simulink model "model_graphicSim_OnlyDist"  (R2022a)
settings: Solver=FixedStepAuto  StartTime=0.0  StopTime=inf  RelTol=1e-3
values from neighbouring files (symbols this model uses):
  A = 3*3    (= 9)    [Configuration.m]    (also in test_sim.mat; test_sim_10000Ep_v10.mat; test_sim_10000Ep_v12_G_oldScen.mat; test_sim_10000Ep_v1_dist.mat)
  d = A*N*nCells    (= 699840)    [Configuration.m]    (also in get_features.m = A*N*nCells; test_sim.mat = 18432; test_sim_10000Ep_v10.mat; test_sim_10000Ep_v12_G_oldScen.mat)
  egoID = 1    [Configuration.m]    (also in test_sim.mat; test_sim_10000Ep_v10.mat; test_sim_10000Ep_v12_G_oldScen.mat; test_sim_10000Ep_v1_dist.mat)
  frontDistCG = 3.7    [Configuration.m]    (also in test_sim_10000Ep_v10.mat; test_sim_10000Ep_v12_G_oldScen.mat; test_sim_10000Ep_v1_dist.mat; test_sim_1000Ep.mat)
  gridvx = zeros(N, length(TVX))    [construct_tiles.m]    (also in test_sim.mat = [-3.33333333333 -3.21428571429 -3.09523809524 -2.97619047619; test_sim_10000Ep_v10.mat = [-2.8 -2.75555555556 -2.71111111111 -2.66666666667 -2.622222; test_sim_10000Ep_v12_G_oldScen.mat = [-2.8 -2.75555555556 -2.71111111111 -2.66666666667 -2.622222; test_sim_10000Ep_v1_dist.mat = [-2.8 -2.75555555556 -2.71111111111 -2.66666666667 -2.622222)
  gridvy = zeros(N, length(TVY))    [construct_tiles.m]    (also in test_sim.mat = [-3.33333333333 -3.16666666667 -3 -2.83333333333 -2.66666666; test_sim_10000Ep_v10.mat = [-28 -27.3777777778 -26.7555555556 -26.1333333333 -25.511111; test_sim_10000Ep_v12_G_oldScen.mat = [-28 -27.3777777778 -26.7555555556 -26.1333333333 -25.511111; test_sim_10000Ep_v1_dist.mat = [-28 -27.3777777778 -26.7555555556 -26.1333333333 -25.511111)
  gridx = zeros(N, length(TX))    [construct_tiles.m]    (also in test_sim.mat = [-8.33333333333 -8.18452380952 -8.03571428571 -7.8869047619 ; test_sim_10000Ep_v10.mat = [-5 -4.94444444444 -4.88888888889 -4.83333333333 -4.77777777; test_sim_10000Ep_v12_G_oldScen.mat = [-5 -4.94444444444 -4.88888888889 -4.83333333333 -4.77777777; test_sim_10000Ep_v1_dist.mat = [-5 -4.94444444444 -4.88888888889 -4.83333333333 -4.77777777)
  gridy = zeros(N, length(TY))    [construct_tiles.m]    (also in test_sim.mat = [-16.6666666667 -16.3095238095 -15.9523809524 -15.5952380952; test_sim_10000Ep_v10.mat = [-2 -1.93333333333 -1.86666666667 -1.8 -1.73333333333 -1.666; test_sim_10000Ep_v12_G_oldScen.mat = [-2 -1.93333333333 -1.86666666667 -1.8 -1.73333333333 -1.666; test_sim_10000Ep_v1_dist.mat = [0.4 0.453333333333 0.506666666667 0.56 0.613333333333 0.666)
  gridyaw = [-504 -489.6 -475.2 -460.8 -446.4 -432 -417.6 -403.2 -388.8 -374.4 -360 -345.6 ... (70 elements, 10x7)]    [test_sim_10000Ep_v10.mat]    (also in test_sim_10000Ep_v12_G_oldScen.mat; test_sim_10000Ep_v1_dist.mat = [-126 -122.4 -118.8 -115.2 -111.6 -108 -104.4 -100.8 -97.2 -; test_sim_1000Ep.mat = [-600 -570 -540 -510 -480 -450 -420 -390 -360 -330 -300 -270; test_sim_1000Ep_v2newparam.mat = [-600 -570 -540 -510 -480 -450 -420 -390 -360 -330 -300 -270)
  lb_angSt = -900    [Configuration.m]    (also in test_sim_10000Ep_v10.mat = -1080; test_sim_10000Ep_v12_G_oldScen.mat = -1080; test_sim_10000Ep_v1_dist.mat; test_sim_10984Ep_vOld_dist.mat)
  lbvx = -2    [Configuration.m]    (also in test_sim.mat; test_sim_10000Ep_v10.mat; test_sim_10000Ep_v12_G_oldScen.mat; test_sim_10000Ep_v1_dist.mat)
  lbvy = -20    [Configuration.m]    (also in test_sim.mat = -2; test_sim_10000Ep_v10.mat; test_sim_10000Ep_v12_G_oldScen.mat; test_sim_10000Ep_v1_dist.mat)
  lbx = 0    [Configuration.m]    (also in test_sim.mat; test_sim_10000Ep_v10.mat; test_sim_10000Ep_v12_G_oldScen.mat; test_sim_10000Ep_v1_dist.mat)
  lby = 2    [Configuration.m]    (also in test_sim.mat = -10; test_sim_10000Ep_v10.mat = 0; test_sim_10000Ep_v12_G_oldScen.mat = 0; test_sim_10000Ep_v1_dist.mat)
  lbyaw = -90    [Configuration.m]    (also in script_verificaAddestramento.m; test_sim_10000Ep_v1_dist.mat; test_sim_10984Ep_vOld_dist.mat)
  leftDistCG = 0.9    [Configuration.m]    (also in test_sim_10000Ep_v10.mat; test_sim_10000Ep_v12_G_oldScen.mat; test_sim_10000Ep_v1_dist.mat; test_sim_1000Ep.mat)
  M = 5    [Configuration.m]    (also in test_sim.mat = 3; test_sim_10000Ep_v10.mat; test_sim_10000Ep_v12_G_oldScen.mat; test_sim_10000Ep_v1_dist.mat)
  N = 10    [Configuration.m]    (also in test_sim.mat = 8; test_sim_10000Ep_v10.mat; test_sim_10000Ep_v12_G_oldScen.mat; test_sim_10000Ep_v1_dist.mat)
  passo_steerang = 180    [Configuration.m]    (also in test_sim.mat = 30; test_sim_10000Ep_v10.mat; test_sim_10000Ep_v12_G_oldScen.mat; test_sim_10000Ep_v1_dist.mat)
  passo_v = 0.5    [Configuration.m]    (also in test_sim.mat = 0.1; test_sim_10000Ep_v10.mat; test_sim_10000Ep_v12_G_oldScen.mat; test_sim_10000Ep_v1_dist.mat)
  retroDistCG = 1    [Configuration.m]    (also in test_sim_10000Ep_v10.mat; test_sim_10000Ep_v12_G_oldScen.mat; test_sim_10000Ep_v1_dist.mat; test_sim_1000Ep.mat)
  s = sp    [graphicSimulation2D.m]
  safetyDist = 0.5    [Configuration.m]    (also in test_sim.mat = 1.5; test_sim_10000Ep_v10.mat = 1; test_sim_10000Ep_v12_G_oldScen.mat = 1; test_sim_10000Ep_v1_dist.mat)
  Ts = 0.1    [Configuration.m]    (also in test_sim_10000Ep_v10.mat; test_sim_10000Ep_v12_G_oldScen.mat; test_sim_10000Ep_v1_dist.mat; test_sim_1000Ep.mat)
  ub_angSt = 900    [Configuration.m]    (also in test_sim_10000Ep_v10.mat = 1080; test_sim_10000Ep_v12_G_oldScen.mat = 1080; test_sim_10000Ep_v1_dist.mat; test_sim_10984Ep_vOld_dist.mat)
  ubvx = 2    [Configuration.m]    (also in test_sim.mat; test_sim_10000Ep_v10.mat; test_sim_10000Ep_v12_G_oldScen.mat; test_sim_10000Ep_v1_dist.mat)
  ubvy = 20    [Configuration.m]    (also in test_sim.mat = 2; test_sim_10000Ep_v10.mat; test_sim_10000Ep_v12_G_oldScen.mat; test_sim_10000Ep_v1_dist.mat)
  ubx = 25    [Configuration.m]    (also in test_sim.mat; test_sim_10000Ep_v10.mat; test_sim_10000Ep_v12_G_oldScen.mat; test_sim_10000Ep_v1_dist.mat)
  uby = 10    [Configuration.m]    (also in test_sim.mat; test_sim_10000Ep_v10.mat; test_sim_10000Ep_v12_G_oldScen.mat; test_sim_10000Ep_v1_dist.mat)
  ubyaw = 90    [Configuration.m]    (also in script_verificaAddestramento.m; test_sim_10000Ep_v1_dist.mat; test_sim_10984Ep_vOld_dist.mat)
  w = zeros(d, 1)    [Configuration.m]    (also in test_sim.mat = [0 0 0 0 0 0 0 0 0 0 0 0 ... (18432 elements, 18432x1)]; test_sim_10000Ep_v10.mat = [0 0 0 0 0 0 0 0 0 0 0 0 ... (699840 elements, 699840x1)]; test_sim_10000Ep_v12_G_oldScen.mat = [0 0 0 0 0 0 0 0 0 0 0 0 ... (699840 elements, 699840x1)]; test_sim_10000Ep_v1_dist.mat = [0 0 0 0 0 0 0 0 0 0 0 0 ... (699840 elements, 699840x1)])
  x_0 = 20*rand+2    [Configuration.m]    (also in script_verificaAddestramento.m = s(1))
  y_0 = -(3*rand+2.2)    [Configuration.m]    (also in script_verificaAddestramento.m = -s(2))
undefined symbols (not defined in the file or in its folder): deg, driving, rad
libraries: drivingscenarioandsensors x17, simulink_extras x2, sim3dlib x1, sim3dautolib x1, aerolibconvert2 x1, vehdynlibsteering x1, autolibshared x1
(part 1 of 6)
settings Model: Creator=User  LastModifiedBy=User

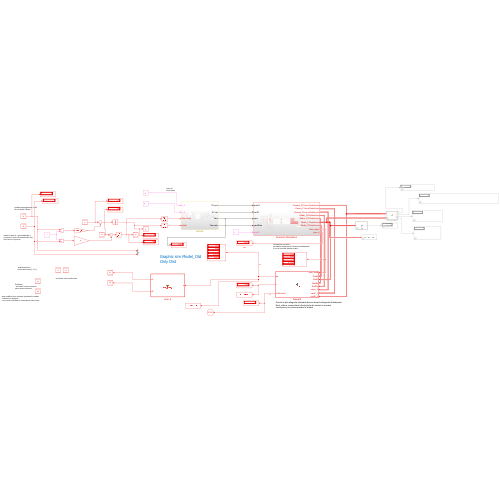
[thumbnail: Simulink's stored preview of the top-level diagram]
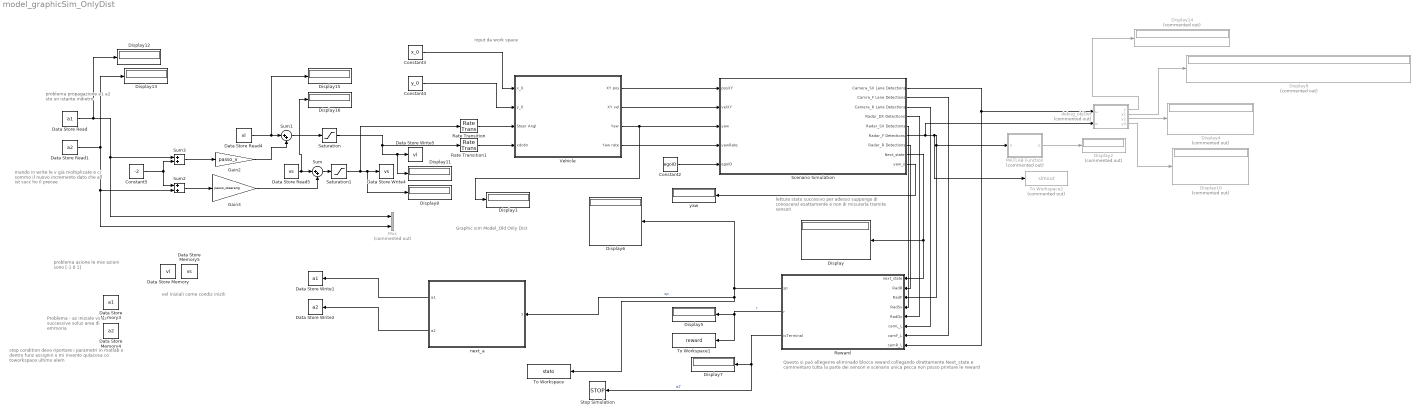
== system model_graphicSim_OnlyDist ==
  note: Questo si può allegerire eliminado blocco reward collegando direttamente
      | Next_state e commentaro tutta la parte dei sensori e scenario
      | unica pecca non posso printare le reward
  note: mando in write le v già moltiplicate e
      | ci sommo il nuovo incremento dato che
      | all ist succ ho il precee
  note: problema azione
      | le mie azioni sono [-1 0 1]
  note: vel iniziali come condiz inizili
  note: stop condition devo riportare i parametri in matlab
      | o dentro funz assignin
      | o mi invento qulacosa co toworkspace ultimo elem
  note: Problema
      | - az iniziale vs az successive
      | soluz area di emmoria
  note: problema propagazione a1 a2
      | sto un istante indietro
  note: input da work space
  note: Graphic sim Model_Old
      | Only Dist
  note: lettura stato succesivo
      | per adesso suppongo di conosceral esattamente
      | e non di misurarla tramite sensori
  Constant2 : Constant  Value=egoID
  Constant3 : Constant  Value=x_0
  Constant4 : Constant  Value=y_0
  Constant5 : Constant  Value=-2
  Data Store Memory : DataStoreMemory  DataStoreName=vl  WriteAfterWriteMsg=warning  ShowAdditionalParam=off
  Data Store Memory3 : DataStoreMemory  DataStoreName=a1  WriteAfterWriteMsg=warning  InitialValue=az_1  VectorParams1D=off  ShowAdditionalParam=off  OutDataTypeStr=double
  Data Store Memory4 : DataStoreMemory  DataStoreName=a2  WriteAfterWriteMsg=warning  InitialValue=az_2  VectorParams1D=off  ShowAdditionalParam=off  OutDataTypeStr=double
  Data Store Memory5 : DataStoreMemory  DataStoreName=vs  WriteAfterWriteMsg=warning  ShowAdditionalParam=off
  Data Store Read : DataStoreRead  DataStoreName=a1  IndexOptions=Index vector (dialog)  Indices=1  OutputSizes=1
  Data Store Read1 : DataStoreRead  DataStoreName=a2  IndexOptions=Index vector (dialog)  Indices=1  OutputSizes=1
  Data Store Read4 : DataStoreRead  DataStoreName=vl  IndexOptions=Index vector (dialog)  Indices=1  OutputSizes=1
  Data Store Read5 : DataStoreRead  DataStoreName=vs  IndexOptions=Index vector (dialog)  Indices=1  OutputSizes=1
  Data Store Write1 : DataStoreWrite  DataStoreName=a1  IndexOptions=Index vector (dialog)  Indices=1  OutputSizes=1
  Data Store Write2 : DataStoreWrite  DataStoreName=a2  IndexOptions=Index vector (dialog)  Indices=1  OutputSizes=1
  Data Store Write4 : DataStoreWrite  DataStoreName=vs  IndexOptions=Index vector (dialog)  Indices=1  OutputSizes=1
  Data Store Write5 : DataStoreWrite  DataStoreName=vl  IndexOptions=Index vector (dialog)  Indices=1  OutputSizes=1
  Display{,1,5..8,11..13,15..16} (11 alike) : Display
  Display{2,4,9..10,14} (5 alike) : Display  Commented=on
  Gain2 : Gain  Gain=passo_v
  Gain3 : Gain  Gain=passo_steerang
  MATLAB Function : MATLAB Function  Commented=on  TreatAsAtomicUnit=on
  Mux : Mux  Commented=on  Inputs=2
  Rate Transition : RateTransition
  Rate Transition1 : RateTransition
  Reward : MATLAB Function  TreatAsAtomicUnit=on
  Saturation : Saturate  UpperLimit=ubvx  LowerLimit=lbvx
  Saturation1 : Saturate  UpperLimit=ub_angSt  LowerLimit=lb_angSt
  Scenario Simulation : Subsystem
  Stop Simulation : Stop
  Sum : Sum  Inputs=|++
  Sum1 : Sum  Inputs=|++
  Sum2 : Sum
  Sum3 : Sum
  To Workspace : ToWorkspace  VariableName=stato  SampleTime=-1
  To Workspace1 : ToWorkspace  VariableName=reward  SampleTime=-1
  To Workspace2 : ToWorkspace  Commented=on  VariableName=simout  SaveFormat=Timeseries  SampleTime=-1
  Vehicle : Subsystem
  debug_objDet : MATLAB Function  Commented=on  TreatAsAtomicUnit=on
  next_a : MATLAB Function  TreatAsAtomicUnit=on
  yaw : Display
  wires:
  Saturation1/1 -> Rate Transition/1, Display8/1, Data Store Write4/1
  Rate Transition/1 -> Vehicle/3(Steer Angl)
  Reward/2(r) -> To Workspace1/1, Display5/1  "r"
  Vehicle/3(Yaw) -> Display1/1, Scenario Simulation/3(yaw)
  Gain2/1 -> Sum1/2
  Sum3/1 -> Gain2/1
  Data Store Read5/1 -> Display16/1, Sum/1
  Data Store Read/1 -> Display12/1, Sum3/1, Mux/1
  Sum1/1 -> Saturation/1
  Sum/1 -> Saturation1/1
  Sum2/1 -> Gain3/1
  Saturation/1 -> Data Store Write5/1, Display11/1, Rate Transition1/1
  Reward/3(isTerminal) -> Stop Simulation/1, Display7/1  "isT"
  Data Store Read1/1 -> Display13/1, Sum2/2, Mux/2
  Constant5/1 -> Sum3/2, Sum2/1
  Gain3/1 -> Sum/2
  Constant3/1 -> Vehicle/1(x_0)
  Data Store Read4/1 -> Display15/1, Sum1/1
  Reward/1(sp) -> Display6/1, To Workspace/1, next_a/1(s)  "sp"
  Vehicle/4(Yaw rate) -> Scenario Simulation/4(yawRate)
  Constant2/1 -> Scenario Simulation/5(egoID)
  Vehicle/2(XY vel) -> Scenario Simulation/2(velXY)
  Rate Transition1/1 -> Vehicle/4(xdotin)
  Vehicle/1(XY pos) -> Scenario Simulation/1(posXY)
  Constant4/1 -> Vehicle/2(y_0)
  next_a/1(a1) -> Data Store Write1/1
  next_a/2(a2) -> Data Store Write2/1
  Scenario Simulation/7(Radar_R Detections) -> Reward/2(RadR)
  Scenario Simulation/5(" Radar_SX Detections") -> Reward/4(RadSx)
  Scenario Simulation/4(Radar_DX Detections) -> Reward/5(RadDx)
  Scenario Simulation/3(Camera_R Lane Detections) -> Reward/6(camL_L)
  Scenario Simulation/2(" Camra_F Lane Detections") -> Reward/7(camF_L)
  Scenario Simulation/1(Camera_SX Lane Detections) -> debug_objDet/1(u), Reward/8(camR_L)
  Scenario Simulation/8(Next_state) -> Display/1, Reward/1(next_state)
  Scenario Simulation/9(yaw_s) -> yaw/1
  Scenario Simulation/6(Radar_F Detections) -> debug_objDet/2(o), MATLAB Function/1(u), Reward/3(RadF), To Workspace2/1
  MATLAB Function/1(y) -> Display2/1
  debug_objDet/4(y3) -> Display10/1
  debug_objDet/1(y) -> Display14/1
  debug_objDet/3(y2) -> Display4/1
  debug_objDet/2(y1) -> Display9/1

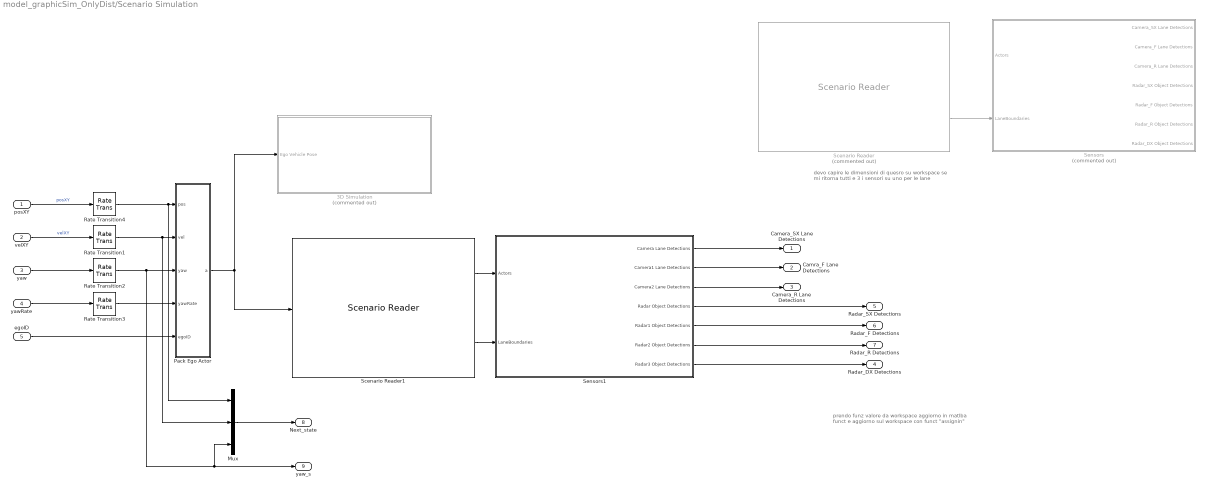
== system model_graphicSim_OnlyDist/Scenario Simulation ==
  note: devo capire le dimensioni di quesro su workspace
      | se mi ritorna tutti e 3 i sensori su uno per le lane
  note: prendo funz valore da workspace
      | aggiorno in matlba funct e aggiorno sul workspace
      | con funct "assignin"
  posXY : Inport
  velXY : Inport  Port=2
  yaw : Inport  Port=3
  yawRate : Inport  Port=4
  egoID : Inport  Port=5
  3D Simulation : Subsystem  Commented=on
  Mux : Mux  Inputs=3
  Pack Ego Actor : MATLAB Function  TreatAsAtomicUnit=on
  Rate Transition{1..4} (4 alike) : RateTransition  OutPortSampleTime=Ts
  Scenario Reader : drivingscenarioandsensors/Scenario Reader  Commented=on  ScenarioSource=From file  ScenarioFileName=C:\Users\User\OneDrive\Desktop\Thesis_Project\project\parking_Scenario_withRadar.mat  ScenarioVariableName=scenario  OutputCoordinateSystem=Vehicle coordinates  EgoVehicleSource=Input port  EgoVehicleActorID=1  OrientVehiclesOnRoad=off  OutputEgoVehiclePose=off  OutputEgoVehicleState=off  SampleTime=Ts  LaneBoundaryOutput=Ego vehicle lane boundaries  LaneBoundaryDistance=linspace(-150, 150, 101)  LaneBoundaryLocation=Center of lane markings  BusNameSource=Auto  BusName=BusActors  BusNumActorsSource=Scenario  BusNumActors=100  BusName2Source=Auto  BusName2=BusLaneBoundaries  BusNumLaneBoundariesSource=Scenario  BusNumLaneBoundaries=10  BusName3Source=Auto  BusName3=BusEgoActor  BusName4Source=Auto  BusName4=BusEgoState  ShowCoordinateLabels=on  SimulateUsing=Interpreted execution
  Scenario Reader1 : drivingscenarioandsensors/Scenario Reader  ScenarioSource=From file  ScenarioFileName=C:\Users\User\OneDrive\Desktop\Thesis_Project\project\parking_Scenario_withRadar_OLD.mat  ScenarioVariableName=scenario  OutputCoordinateSystem=Vehicle coordinates  EgoVehicleSource=Input port  EgoVehicleActorID=1  OrientVehiclesOnRoad=off  OutputEgoVehiclePose=off  OutputEgoVehicleState=off  SampleTime=0.1  LaneBoundaryOutput=Ego vehicle lane boundaries  LaneBoundaryDistance=linspace(-150, 150, 101)  LaneBoundaryLocation=Center of lane markings  BusNameSource=Auto  BusName=BusActors  BusNumActorsSource=Scenario  BusNumActors=100  BusName2Source=Auto  BusName2=BusLaneBoundaries  BusNumLaneBoundariesSource=Scenario  BusNumLaneBoundaries=10  BusName3Source=Auto  BusName3=BusEgoActor  BusName4Source=Auto  BusName4=BusEgoState  ShowCoordinateLabels=on  SimulateUsing=Interpreted execution
  Sensors : Subsystem  Commented=on
  Sensors1 : Subsystem
  Camera_SX Lane Detections : Outport
  " Camra_F Lane Detections" : Outport  Port=2
  Camera_R Lane Detections : Outport  Port=3
  Radar_DX Detections : Outport  Port=4
  " Radar_SX Detections" : Outport  Port=5
  Radar_F Detections : Outport  Port=6
  Radar_R Detections : Outport  Port=7
  Next_state : Outport  Port=8
  yaw_s : Outport  Port=9
  wires:
  Pack Ego Actor/1(a) -> Scenario Reader1/1, 3D Simulation/1(Ego Vehicle Pose)
  Sensors1/5(Radar1 Object Detections) -> Radar_F Detections/1
  yawRate/1 -> Rate Transition3/1
  Rate Transition1/1 -> Mux/2, Pack Ego Actor/2(vel)
  Rate Transition4/1 -> Mux/1, Pack Ego Actor/1(pos)
  Rate Transition3/1 -> Pack Ego Actor/4(yawRate)
  Rate Transition2/1 -> Mux/3, yaw_s/1, Pack Ego Actor/3(yaw)
  egoID/1 -> Pack Ego Actor/5(egoID)
  velXY/1 -> Rate Transition1/1  "velXY"
  posXY/1 -> Rate Transition4/1  "posXY"
  yaw/1 -> Rate Transition2/1
  Sensors1/1(Camera Lane Detections) -> Camera_SX Lane Detections/1
  Sensors1/2(Camera1 Lane Detections) -> " Camra_F Lane Detections"/1
  Sensors1/3(Camera2 Lane Detections) -> Camera_R Lane Detections/1
  Sensors1/4(Radar Object Detections) -> " Radar_SX Detections"/1
  Sensors1/6(Radar2 Object Detections) -> Radar_R Detections/1
  Sensors1/7(Radar3 Object Detections) -> Radar_DX Detections/1
  Mux/1 -> Next_state/1
  Scenario Reader/2 -> Sensors/2(LaneBoundaries)
  Scenario Reader1/1 -> Sensors1/1(Actors)
  Scenario Reader1/2 -> Sensors1/2(LaneBoundaries)

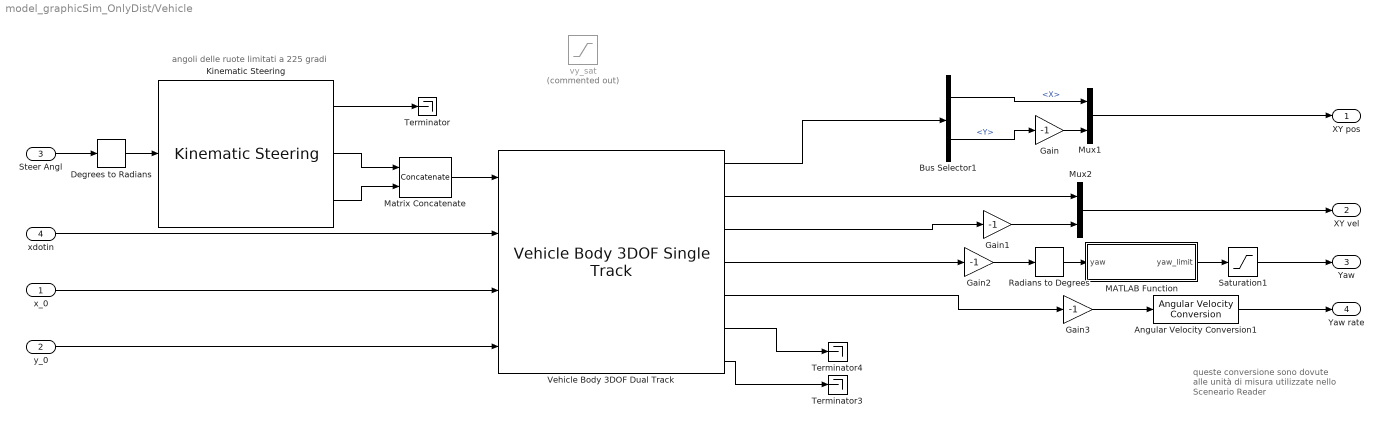
== system model_graphicSim_OnlyDist/Vehicle ==
  note: angoli delle ruote limitati a 225 gradi
  note: queste conversione sono dovute
      | alle unità di misura utilizzate nello
      | Sceneario Reader
  x_0 : Inport
  y_0 : Inport  Port=2
  Steer Angl : Inport  Port=3
  xdotin : Inport  Port=4
  Angular Velocity Conversion1 : aerolibconvert2/Angular Velocity Conversion  IU=rad/s  OU=deg/s
  Bus Selector1 : BusSelector  OutputSignals=InertFrm.Cg.Disp.X,InertFrm.Cg.Disp.Y
  Degrees to Radians : simulink_extras/Transformations/Degrees to Radians
  Gain{,1..3} (4 alike) : Gain  Gain=-1
  Kinematic Steering : vehdynlibsteering/Kinematic Steering  StrgType=Ackerman  StrgRatioType=Constant  Loc=Front  NrmlFctr=0.01  TrckWdth=1  WhlBase=1.524  Db=0  StrgRng=5*pi  StrgAngBpts="[-6.2832   -5.0265   -3.7699   -2.5133   -1.2566         0    1.2566    2.5133    3.7699    5.0265    6.2832]"  StrgRatioTbl=|  StrgRatio=100  PctAckIn=off  PctAck=100  PctAckTbl=ones(1,11)*100  StrgArmLngth=0.1  RckCsLngth=0.5  TieRodLngth=0.248  D=0.2  PnnRadius=0.00085818  PnnRadiusTbl="[0.0055    0.0055    0.0056    0.0057    0.0058    0.0057    0.0057    0.0057    0.0056    0.0055    0.0055]"  RodLngth=0.1  ParaArmLngth=0.9  aMode=2
      | [13.5000   13.3750   13.2500   13.1250   13.0000   13.0000   13.0000   13.1250   13.2500   13.3750   13.5000
      | ]
  MATLAB Function : MATLAB Function  TreatAsAtomicUnit=on
  Matrix Concatenate : Concatenate  ConcatenateDimension=2
  Mux1 : Mux  Inputs=2
  Mux2 : Mux  Inputs=2
  Radians to Degrees : simulink_extras/Transformations/Radians to Degrees
  Saturation1 : Saturate  UpperLimit=360  LowerLimit=-360
  Terminator : Terminator
  Terminator3 : Terminator
  Terminator4 : Terminator
  Vehicle Body 3DOF Dual Track : autolibshared/Vehicle Body 3DOF Single Track  trackMode=Dual  inputMode=External longitudinal velocity  frontSteerMode=on  rearSteerMode=off  windMode=off  muMode=off  extFMode=off  extMMode=off  htchFMode=off  htchMMode=off  extXo=on  extpsio=off  extxdoto=off  extro=off  extYo=on  extTamb=off  extydoto=off  aMode=2  NF=2  NR=2  m=2000  a=1.4  b=1.6  h=0.35  dh=1  hh=0.2  X_o=0  xdot_o=0  CalphaMode=off  sigmaMode=on  d=0  hl=0  w=[1.4,1.4]  Cy_f=12e3  Cy_r=11e3  sigma_f=.1  sigma_r=.1  alpha_f_brk=[-.1 .1]  Cy_f_data=[-9e3 9e3]  alpha_r_brk=[-.1 .1]  Cy_r_data=[-9e3 9e3]  Y_o=0  ydot_o=0  Izz=4000  psi_o=0  r_o=0  Af=2  Cd=.3  Cl=.1  Cpm=.1  beta_w=[0 0.01:0.01:0.3]  Cs=[0:0.03:0.9]  Cym=[0 1e-6:0.01:0.3]  Pabs=101325  Tair=273  g=9.81  mu=1  xdot_tol=.01  Fznom=5000  Fxtire_sat=7e4  Fytire_sat=7e4  longOff=0  latOff=0  vertOff=0  wrapAng=off
      settings: SourceProductBaseCode=PW,DR,MT,VE
  vy_sat : Saturate  Commented=on  UpperLimit=ubvy  LowerLimit=lbvy
  XY pos : Outport
  XY vel : Outport  Port=2
  Yaw : Outport  Port=3
  Yaw rate : Outport  Port=4
  wires:
  Bus Selector1/2 -> Gain/1  "<Y>"
  Kinematic Steering/3 -> Matrix Concatenate/2
  Matrix Concatenate/1 -> Vehicle Body 3DOF Dual Track/1
  Vehicle Body 3DOF Dual Track/6 -> Terminator4/1
  Mux1/1 -> XY pos/1
  Bus Selector1/1 -> Mux1/1  "<X>"
  Kinematic Steering/1 -> Terminator/1
  Degrees to Radians/1 -> Kinematic Steering/1
  Vehicle Body 3DOF Dual Track/7 -> Terminator3/1
  Kinematic Steering/2 -> Matrix Concatenate/1
  Mux2/1 -> XY vel/1
  Steer Angl/1 -> Degrees to Radians/1
  xdotin/1 -> Vehicle Body 3DOF Dual Track/2
  Radians to Degrees/1 -> MATLAB Function/1(yaw)
  Gain3/1 -> Angular Velocity Conversion1/1
  x_0/1 -> Vehicle Body 3DOF Dual Track/3
  y_0/1 -> Vehicle Body 3DOF Dual Track/4
  Vehicle Body 3DOF Dual Track/3 -> Gain1/1
  MATLAB Function/1(yaw_limit) -> Saturation1/1
  Saturation1/1 -> Yaw/1
  Vehicle Body 3DOF Dual Track/2 -> Mux2/1
  Vehicle Body 3DOF Dual Track/1 -> Bus Selector1/1
  Gain/1 -> Mux1/2
  Gain1/1 -> Mux2/2
  Gain2/1 -> Radians to Degrees/1
  Vehicle Body 3DOF Dual Track/5 -> Gain3/1
  Vehicle Body 3DOF Dual Track/4 -> Gain2/1
  Angular Velocity Conversion1/1 -> Yaw rate/1

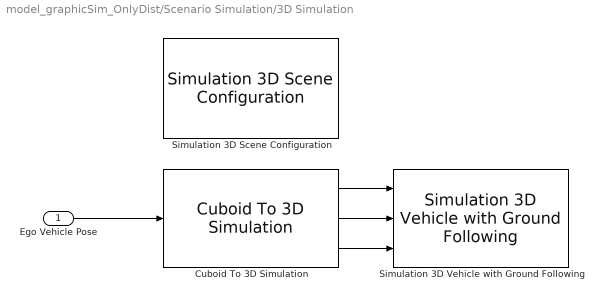
== system model_graphicSim_OnlyDist/Scenario Simulation/3D Simulation ==
  Ego Vehicle Pose : Inport
  Cuboid To 3D Simulation : drivingscenarioandsensors/Cuboid To 3D Simulation  SpecifyActorID=on  ActorIDToConvert=1  SimulateUsing=Interpreted execution
      settings: SourceProductBaseCode=DR
  Simulation 3D Scene Configuration : sim3dlib/Simulation 3D Scene Configuration  Priority=0  ProjectFormat=Default Scenes  SceneDesc=Straight road  ProjectName=C:\Program Files\MATLAB\R2022a\toolbox\shared\sim3d_projects\automotive_project\UE4\WindowsNoEditor\VehicleSimulation.exe  ScenePath=/Game/Maps/HwStrght  vehTagList={'Scene Origin';'SimulinkVehicle1'}  vehTag=SimulinkVehicle1  OpVisEn=off  Ts=1/60  EnableWindow=on  EnableRemoteAccess=off  EnableWeather=off  SunAltitude=40.0  SunAzimuth=90  clouds=10  wind=1  fog=0  rain=0  sensorTag=MainCamera1  sensorId=1  sensorName=MainCamera1  mountLoc=Origin  offsetFlag=off  tmountOffset=[0, 0, 0]  rmountOffset=[0, 0, 0]  HorizontalResolution=1280  VerticalResolution=720  HorizontalFOV=60  mountPoint=[0 0 0]  mountOrientation=[0 0 0]  aMode=3  ID=1
      settings: SourceProductBaseCode=VE,AE,DR,UV,VE
  Simulation 3D Vehicle with Ground Following : sim3dautolib/Simulation 3D Vehicle with Ground Following  Priority=-1  PassVehMesh=Muscle car  MeshPath=/MathWorksSimulation/Vehicles/Muscle/Meshes/SK_MuscleCar.SK_MuscleCar  TrackWidth=1.9  WheelBase=3  WheelRadius=0.35  VehColor=Red  InitialPos=[0, 0, 0]  InitialRot=[0, 0, 0]  ActorName=SimulinkVehicle1  SampleTime=-1  ActorType=SimulinkVehicle  ID=1  aMode=3  ActorTag=SimulinkVehicle1  CoordinateScheme=ISO  VehLightsControl=off  HeadlightColor=[ 1, 1, 1 ]  HighBeamIntensity=100000  LowBeamIntensity=60000  HighBeamConeAngle=70  LowBeamConeAngle=70  LeftHeadlightOrientation=[ 0, 0 ]  RightHeadlightOrientation=[ 0, 0 ]  BrakelightIntensity=500  ReverselightIntensity=500  SignallightIntensity=500  SignallightPeriod=1  SignalPulseWidth=50  TransformOutportEnabled=off
      settings: SourceProductBaseCode=VE,AE,DR,UV,VE
  wires:
  Cuboid To 3D Simulation/3 -> Simulation 3D Vehicle with Ground Following/3
  Cuboid To 3D Simulation/2 -> Simulation 3D Vehicle with Ground Following/2
  Cuboid To 3D Simulation/1 -> Simulation 3D Vehicle with Ground Following/1
  Ego Vehicle Pose/1 -> Cuboid To 3D Simulation/1
